simulink model "OP_simulink"  (R2023b)
settings: Solver=VariableStepAuto  StartTime=0.0  StopTime=10.0  RelTol=1e-3
values from neighbouring files (symbols this model uses):
  A = [0 1;0 (R1*R3*C2)/(R1*R2*R3*C1*C2)]    [datos_simulink.m]
  B = [0;(R2)/(R1*R2*R3*C1*C2)]    [datos_simulink.m]
  C1 = 1e-6    (= 1e-06)    [datos_simulink.m]    (also in sistema_op.m)
  C2 = 1e-6    (= 1e-06)    [datos_simulink.m]    (also in sistema_op.m)
  R1 = 5000000    [datos_simulink.m]    (also in sistema_op.m)
  R2 = 5000000    [datos_simulink.m]    (also in sistema_op.m)
  R3 = 5000000    [datos_simulink.m]    (also in sistema_op.m)
settings Model: Creator=Envy  LastModifiedBy=Envy

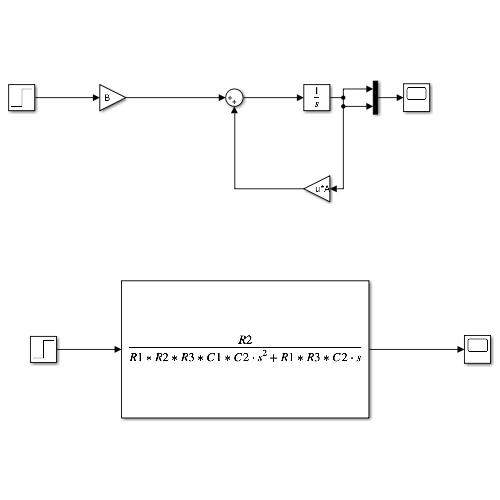
[thumbnail: Simulink's stored preview of the top-level diagram]
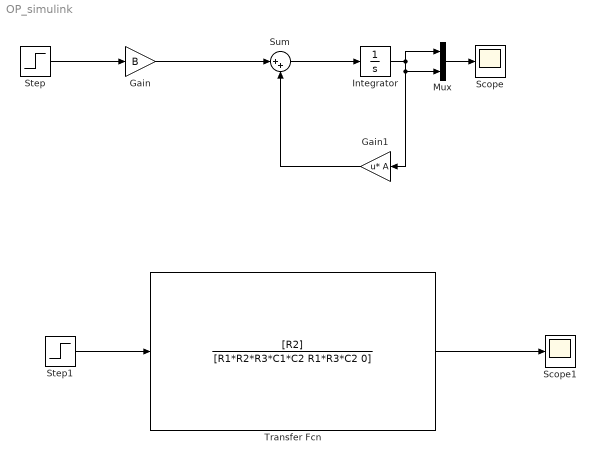
== system OP_simulink ==
  Gain : Gain  Gain=B
  Gain1 : Gain  Gain=A  Multiplication=Matrix(u*K)
  Integrator : Integrator
  Mux : Mux  Inputs=2
  Scope : Scope
  Scope1 : Scope
  Step : Step  Time=0  After=12  SampleTime=0
  Step1 : Step  Time=0  After=12  SampleTime=0
  Sum : Sum  Inputs=|++
  Transfer Fcn : TransferFcn  Numerator=[R2]  Denominator=[R1*R2*R3*C1*C2 R1*R3*C2 0]
  wires:
  Gain/1 -> Sum/1
  Sum/1 -> Integrator/1
  Integrator/1 -> Gain1/1, Mux/2, Mux/1
  Gain1/1 -> Sum/2
  Step/1 -> Gain/1
  Mux/1 -> Scope/1
  Transfer Fcn/1 -> Scope1/1
  Step1/1 -> Transfer Fcn/1
